simulink model "FOC_SMPMSM_SPWM"  (R2020b)
settings: Solver=FixedStepDiscrete  StartTime=0.0  StopTime=2  RelTol=1e-3
undefined symbols (not defined in the file): Kp_speed, Lq, PM_flux, pp, Rs
libraries: powerlib x23, simulink x5, pid_lib x3, powerlib_meascontrol x1
settings Model: SimulationMode=accelerator  Creator=ryusl  LastModifiedBy=90554
settings DataIOCC: SaveFormat=Array  ReturnWorkspaceOutputs=off
settings SFSimCC: CustomCodeUndefinedFunction=UseInterfaceOnly

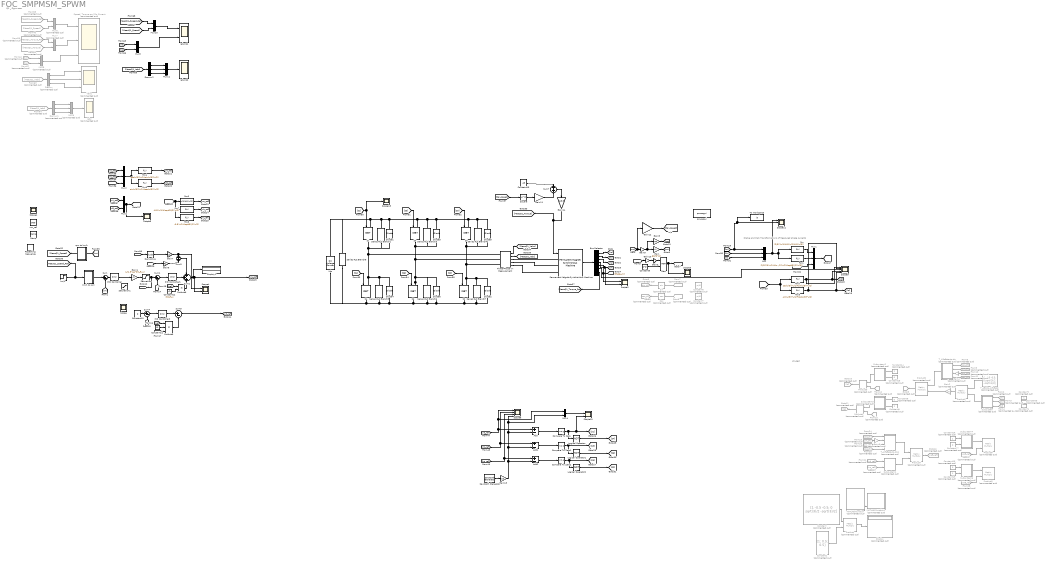
== system FOC_SMPMSM_SPWM ==
  note: Q1 _ Figures
  note: Unused
  note: Clarke and Park Transformations of Measured phase currents
  Add : Sum  Inputs=+-
  Add1 : Sum  Inputs=+-
  Add2 : Sum  Inputs=+-
  Bus Selector : BusSelector  OutputSignals=Stator current is_a (A),Stator current is_b (A),Stator current is_c (A),Rotor speed wm (rad/s),Rotor angle thetam (rad),Stator current is_d (A),Electromagnetic torque Te (N*m)
  Compare To Zero : simulink/Logic and Bit Operations/Compare To Zero  relop=>=  OutDataTypeStr=boolean
  Compare To Zero1 : simulink/Logic and Bit Operations/Compare To Zero  relop=>=  OutDataTypeStr=boolean
  Compare To Zero2 : simulink/Logic and Bit Operations/Compare To Zero  relop=>=  OutDataTypeStr=boolean
  Constant : Constant  Commented=on  Value=[1 -0.5 -0.5; 0 sqrt(3)/2 -sqrt(3)/2]  VectorParams1D=off
  Constant1 : Constant  Commented=on  Value=[1; 0.5; 0.5]  VectorParams1D=off
  Constant10 : Constant  Value=0
  Constant11 : Constant  Value=Lq
  Constant12 : Constant  Value=PM_flux
  Constant13 : Constant  Value=45
  Constant{2,9,14,16,19} (5 alike) : Constant  Commented=on
  Constant{8,15,17..18} (4 alike) : Constant  Commented=on  Value=0
  Constant3 : Constant  Commented=on  Value=-0.5
  Constant4 : Constant  Commented=on  Value=-0.5
  Constant5 : Constant  Value=2*pi
  Constant6 : Constant  Commented=on  Value=pi/6
  Constant7 : Constant  Commented=on  Value=pi/6
  Cos : Trigonometry  Commented=on  Operator=cos
  Demux : Demux  Commented=on  Outputs=3
  Demux1 : Demux  Commented=on  Outputs=3
  Demux2 : Demux  Outputs=3
  Derivative : Derivative
  Diode{1..6} (6 alike) : powerlib/Power Electronics/Diode  Ron=0.001  Lon=0  Vf=0.8  IC=0  UseSnubber=0  Rs=inf  Cs=0  Measurements=off
  Display : Display  Commented=on
  Display1 : Display
  Fcn : Fcn  Expr=(2/3)*(u(1)-0.5*u(2)-0.5*u(3))
  Fcn1 : Fcn  Expr=(2/3)*(0*u(1)+(sqrt(3)/2)*u(2)-(sqrt(3)/2)*u(3))
  Fcn2 : Fcn  Expr=cos(u(3))*u(1)+sin(u(3))*u(2)
  Fcn3 : Fcn  Expr=-sin(u(3))*u(1)+cos(u(3))*u(2)
  Fcn4 : Fcn  Expr=cos(u(3))*u(1)-sin(u(3))*u(2)
  Fcn5 : Fcn  Expr=sin(u(3))*u(1)+cos(u(3))*u(2)
  Fcn6 : Fcn  Expr=u(1)+0*u(2)
  Fcn7 : Fcn  Expr=-0.5*u(1)+(sqrt(3)/2)*u(2)
  Fcn8 : Fcn  Expr=-0.5*u(1)-(sqrt(3)/2)*u(2)
  From{9..10,23,26} (4 alike) : From  Commented=on  GotoTag=sin_th
  From{8,11,24..25} (4 alike) : From  Commented=on  GotoTag=cos_th
  From12 : From  Commented=on  GotoTag=idq
  From13 : From  Commented=on  GotoTag=idq
  From2 : From  Commented=on  GotoTag=ia
  From21 : From  Commented=on  GotoTag=vd_ref
  From22 : From  Commented=on  GotoTag=vq_ref
  From27 : From  Commented=on  GotoTag=vaB_ref
  From28 : From  Commented=on  GotoTag=vaB_ref
  From3 : From  Commented=on  GotoTag=ib
  From4 : From  Commented=on  GotoTag=ic
  From40 : From  Commented=on  GotoTag=MeasQ1_Speed
  From58 : From  Commented=on  GotoTag=MeasQ1_Speed_Ref
  From59 : From  Commented=on  GotoTag=MeasQ1_Torque_Ref
  From6 : From  Commented=on  GotoTag=theta_e
  From60 : From  Commented=on  GotoTag=MeasQ1_Torque
  From61 : From  Commented=on  GotoTag=id
  From62 : From  Commented=on  GotoTag=iq
  From63 : From  Commented=on  GotoTag=MeasQ1_Vabc
  From64 : From  Commented=on  GotoTag=MeasQ1_Iabc
  From7 : From  Commented=on  GotoTag=theta_e
  Gain : Gain  Gain=60/(2*pi)
  Gain1 : Gain  Gain=1/(1.5*pp*PM_flux)
  Gain10 : Gain
  Gain11 : Gain  Gain=0.105
  Gain12 : Gain  Gain=0.3/8.5
  Gain13 : Gain  Gain=210
  Gain14 : Gain  Gain=1/8.5
  Gain2 : Gain  Commented=on  Gain=2/3
  Gain3 : Gain  Gain=pp
  Gain4 : Gain  Commented=on  Gain=-1
  Gain5 : Gain  Gain=pp
  Gain6 : Gain  Gain=Rs
  Gain7 : Gain  Gain=Lq
  Gain8 : Gain  Commented=on  Gain=-1
  Gain9 : Gain
  Goto10 : Goto  Commented=on  GotoTag=id
  Goto11 : Goto  Commented=on  GotoTag=iq
  Goto16 : Goto  Commented=on  GotoTag=vaB_ref
  Goto6 : Goto  Commented=on  GotoTag=cos_th
  Goto8 : Goto  Commented=on  GotoTag=sin_th
  Goto9 : Goto  Commented=on  GotoTag=idq
  Iabc : Scope  Commented=on
  Iabc Q1 : Scope  NumInputPorts=2
  Iabc Q2 : Scope
  Logical Operator : Logic  Operator=NOT  AllPortsSameDT=off  OutDataTypeStr=boolean
  Logical Operator1 : Logic  Operator=NOT  AllPortsSameDT=off  OutDataTypeStr=boolean
  Logical Operator2 : Logic  Operator=NOT  AllPortsSameDT=off  OutDataTypeStr=boolean
  MATLAB Function : MATLAB Function  Commented=on  TreatAsAtomicUnit=on
  MATLAB Function1 : MATLAB Function  Commented=on  TreatAsAtomicUnit=on
  Mux{,1..2,11} (4 alike) : Mux  Inputs=3
  Mux{3..4,8,10} (4 alike) : Mux  Inputs=2
  Mux5 : Mux  Commented=on  Inputs=2
  Mux6 : Mux  Commented=on  Inputs=2
  Mux7 : Mux  Commented=on  Inputs=2
  Mux9 : Mux  Commented=on  Inputs=3
  PID Controller : pid_lib/PID Controller  Controller=PI  Form=Parallel  TimeDomain=Discrete-time  UseExternalTs=off  SampleTime=-1  IntegratorMethod=Forward Euler  FilterMethod=Forward Euler  ControllerParametersSource=internal  P=Kp_speed  I=2  D=0  UseFilter=on  N=100  TunerSelectOption=Transfer Function Based (PID Tuner App)  InitialConditionSource=internal  InitialConditionForIntegrator=0  InitialConditionForFilter=0  DifferentiatorICPrevScaledInput=0  ExternalReset=none  TrackingMode=off  Kt=1  LimitOutput=off  SatLimitsSource=internal  UpperSaturationLimit=inf  LowerSaturationLimit=-inf  LinearizeAsGain=on  AntiWindupMode=none  Kb=1  POutMin=[]  POutMax=[]  IOutMin=[]  IOutMax=[]  DOutMin=[]  DOutMax=[]  NOutMin=[]  NOutMax=[]  SumOutMin=[]  SumOutMax=[]  SaturationOutMin=[]  SaturationOutMax=[]  PParamMin=[]  PParamMax=[]  IParamMin=[]  IParamMax=[]  DParamMin=[]  DParamMax=[]  NParamMin=[]  NParamMax=[]  KbParamMin=[]  KbParamMax=[]  KtParamMin=[]  KtParamMax=[]  KbOutMin=[]  KbOutMax=[]  KtOutMin=[]  KtOutMax=[]  IntegratorOutMin=[]  IntegratorOutMax=[]  FilterOutMin=[]  FilterOutMax=[]  SumI1OutMin=[]  SumI1OutMax=[]  SumI2OutMin=[]  SumI2OutMax=[]  SumI3OutMin=[]  SumI3OutMax=[]  SumI4OutMin=[]  SumI4OutMax=[]  SumDOutMin=[]  SumDOutMax=[]  DifferentiatorOutMin=[]  DifferentiatorOutMax=[]  FilterDiffOutCoefMin=[]  FilterDiffOutCoefMax=[]  ReciprocalOutMin=[]  ReciprocalOutMax=[]  SumDenOutMin=[]  SumDenOutMax=[]  SumNumOutMin=[]  SumNumOutMax=[]  DivideOutMin=[]  DivideOutMax=[]  UdiffTsProdOutMin=[]  UdiffTsProdOutMax=[]  NTsProdOutMin=[]  NTsProdOutMax=[]  UintegralTsProdOutMin=[]  UintegralTsProdOutMax=[]  UngainTsProdOutMin=[]  UngainTsProdOutMax=[]  IntegratorContinuousStateAttributes=''  IntegratorStateMustResolveToSignalObject=off  IntegratorRTWStateStorageClass=Auto  FilterContinuousStateAttributes=''  FilterStateMustResolveToSignalObject=off  FilterRTWStateStorageClass=Auto  ParallelPVariant=InternalParameters  IdealPVariant=Disabled  IVariant=InternalParameters  DVariant=Disabled  IntegratorVariant=Discrete  SatVariant=Disabled  AWVariant=Passthrough  PCopyVariant=Disabled  TRVariant=Disabled  FdbkBlocksVariant=Forward  IdealPFdbkVariant=Disabled  SatFdbkVariant=Disabled  DerivativeFilterVariant=Disabled  NVariant=Disabled  NCopyVariant=Disabled_SignalSpec  FilterICVariant=Disabled  IntegratorICVariant=InternalICs  ExternalResetVariant=Disabled  TRSumVariant=Passthrough  SumFdbkVariant=Disabled  SumVariant=Sum_PI  TsampFilterVariant=InternalTs  TsampNgainVariant=Passthrough  TsampIntegralVariant=Passthrough  ExternalSaturationOutDataTypeStr=Inherit: Same as second input
  PID Controller1 : pid_lib/PID Controller  Controller=PI  Form=Parallel  TimeDomain=Discrete-time  UseExternalTs=off  SampleTime=-1  IntegratorMethod=Forward Euler  FilterMethod=Forward Euler  ControllerParametersSource=internal  P=10  I=1  D=0  UseFilter=on  N=100  TunerSelectOption=Transfer Function Based (PID Tuner App)  InitialConditionSource=internal  InitialConditionForIntegrator=0  InitialConditionForFilter=0  DifferentiatorICPrevScaledInput=0  ExternalReset=none  TrackingMode=off  Kt=1  LimitOutput=off  SatLimitsSource=internal  UpperSaturationLimit=inf  LowerSaturationLimit=-inf  LinearizeAsGain=on  AntiWindupMode=none  Kb=1  POutMin=[]  POutMax=[]  IOutMin=[]  IOutMax=[]  DOutMin=[]  DOutMax=[]  NOutMin=[]  NOutMax=[]  SumOutMin=[]  SumOutMax=[]  SaturationOutMin=[]  SaturationOutMax=[]  PParamMin=[]  PParamMax=[]  IParamMin=[]  IParamMax=[]  DParamMin=[]  DParamMax=[]  NParamMin=[]  NParamMax=[]  KbParamMin=[]  KbParamMax=[]  KtParamMin=[]  KtParamMax=[]  KbOutMin=[]  KbOutMax=[]  KtOutMin=[]  KtOutMax=[]  IntegratorOutMin=[]  IntegratorOutMax=[]  FilterOutMin=[]  FilterOutMax=[]  SumI1OutMin=[]  SumI1OutMax=[]  SumI2OutMin=[]  SumI2OutMax=[]  SumI3OutMin=[]  SumI3OutMax=[]  SumI4OutMin=[]  SumI4OutMax=[]  SumDOutMin=[]  SumDOutMax=[]  DifferentiatorOutMin=[]  DifferentiatorOutMax=[]  FilterDiffOutCoefMin=[]  FilterDiffOutCoefMax=[]  ReciprocalOutMin=[]  ReciprocalOutMax=[]  SumDenOutMin=[]  SumDenOutMax=[]  SumNumOutMin=[]  SumNumOutMax=[]  DivideOutMin=[]  DivideOutMax=[]  UdiffTsProdOutMin=[]  UdiffTsProdOutMax=[]  NTsProdOutMin=[]  NTsProdOutMax=[]  UintegralTsProdOutMin=[]  UintegralTsProdOutMax=[]  UngainTsProdOutMin=[]  UngainTsProdOutMax=[]  IntegratorContinuousStateAttributes=''  IntegratorStateMustResolveToSignalObject=off  IntegratorRTWStateStorageClass=Auto  FilterContinuousStateAttributes=''  FilterStateMustResolveToSignalObject=off  FilterRTWStateStorageClass=Auto  ParallelPVariant=InternalParameters  IdealPVariant=Disabled  IVariant=InternalParameters  DVariant=Disabled  IntegratorVariant=Discrete  SatVariant=Disabled  AWVariant=Passthrough  PCopyVariant=Disabled  TRVariant=Disabled  FdbkBlocksVariant=Forward  IdealPFdbkVariant=Disabled  SatFdbkVariant=Disabled  DerivativeFilterVariant=Disabled  NVariant=Disabled  NCopyVariant=Disabled_SignalSpec  FilterICVariant=Disabled  IntegratorICVariant=InternalICs  ExternalResetVariant=Disabled  TRSumVariant=Passthrough  SumFdbkVariant=Disabled  SumVariant=Sum_PI  TsampFilterVariant=InternalTs  TsampNgainVariant=Passthrough  TsampIntegralVariant=Passthrough  ExternalSaturationOutDataTypeStr=Inherit: Same as second input
  PID Controller2 : pid_lib/PID Controller  Controller=PI  Form=Parallel  TimeDomain=Discrete-time  UseExternalTs=off  SampleTime=-1  IntegratorMethod=Forward Euler  FilterMethod=Forward Euler  ControllerParametersSource=internal  P=10  I=1  D=0  UseFilter=on  N=100  TunerSelectOption=Transfer Function Based (PID Tuner App)  InitialConditionSource=internal  InitialConditionForIntegrator=0  InitialConditionForFilter=0  DifferentiatorICPrevScaledInput=0  ExternalReset=none  TrackingMode=off  Kt=1  LimitOutput=off  SatLimitsSource=internal  UpperSaturationLimit=inf  LowerSaturationLimit=-inf  LinearizeAsGain=on  AntiWindupMode=none  Kb=1  POutMin=[]  POutMax=[]  IOutMin=[]  IOutMax=[]  DOutMin=[]  DOutMax=[]  NOutMin=[]  NOutMax=[]  SumOutMin=[]  SumOutMax=[]  SaturationOutMin=[]  SaturationOutMax=[]  PParamMin=[]  PParamMax=[]  IParamMin=[]  IParamMax=[]  DParamMin=[]  DParamMax=[]  NParamMin=[]  NParamMax=[]  KbParamMin=[]  KbParamMax=[]  KtParamMin=[]  KtParamMax=[]  KbOutMin=[]  KbOutMax=[]  KtOutMin=[]  KtOutMax=[]  IntegratorOutMin=[]  IntegratorOutMax=[]  FilterOutMin=[]  FilterOutMax=[]  SumI1OutMin=[]  SumI1OutMax=[]  SumI2OutMin=[]  SumI2OutMax=[]  SumI3OutMin=[]  SumI3OutMax=[]  SumI4OutMin=[]  SumI4OutMax=[]  SumDOutMin=[]  SumDOutMax=[]  DifferentiatorOutMin=[]  DifferentiatorOutMax=[]  FilterDiffOutCoefMin=[]  FilterDiffOutCoefMax=[]  ReciprocalOutMin=[]  ReciprocalOutMax=[]  SumDenOutMin=[]  SumDenOutMax=[]  SumNumOutMin=[]  SumNumOutMax=[]  DivideOutMin=[]  DivideOutMax=[]  UdiffTsProdOutMin=[]  UdiffTsProdOutMax=[]  NTsProdOutMin=[]  NTsProdOutMax=[]  UintegralTsProdOutMin=[]  UintegralTsProdOutMax=[]  UngainTsProdOutMin=[]  UngainTsProdOutMax=[]  IntegratorContinuousStateAttributes=''  IntegratorStateMustResolveToSignalObject=off  IntegratorRTWStateStorageClass=Auto  FilterContinuousStateAttributes=''  FilterStateMustResolveToSignalObject=off  FilterRTWStateStorageClass=Auto  ParallelPVariant=InternalParameters  IdealPVariant=Disabled  IVariant=InternalParameters  DVariant=Disabled  IntegratorVariant=Discrete  SatVariant=Disabled  AWVariant=Passthrough  PCopyVariant=Disabled  TRVariant=Disabled  FdbkBlocksVariant=Forward  IdealPFdbkVariant=Disabled  SatFdbkVariant=Disabled  DerivativeFilterVariant=Disabled  NVariant=Disabled  NCopyVariant=Disabled_SignalSpec  FilterICVariant=Disabled  IntegratorICVariant=InternalICs  ExternalResetVariant=Disabled  TRSumVariant=Passthrough  SumFdbkVariant=Disabled  SumVariant=Sum_PI  TsampFilterVariant=InternalTs  TsampNgainVariant=Passthrough  TsampIntegralVariant=Passthrough  ExternalSaturationOutDataTypeStr=Inherit: Same as second input
  Permanent Magnet Synchronous Machine : powerlib/Machines/Permanent Magnet Synchronous Machine  NbPhases=3  FluxDistribution=Sinusoidal  RotorType=Round  MechanicalLoad=Torque Tm  PresetModel=No  ShowDetailedParameters=on  MeasurementBus=off  Resistance=Rs  Inductance=8.5e-3  dqInductances=[8.5e-3,8.5e-3]  La=Ld  MachineConstant=Flux linkage established by magnets (V.s)  Flux=PM_flux  VoltageCst=79.8072  TorqueCst=0.66  Flat=120  Mechanical=[2.4232 0 4 0]  PolePairs=4  InitialConditions=[(40*8.5)/(3.6*0.3),0, 0,0]  InitialConditions5ph=[0 0 0 0 0 0]  RefAngle=Aligned with phase A axis (original Park)  IterativeDiscreteModel=Trapezoidal non iterative  TsBlock=1e-6  TsPowergui=0
  Product{,1..4,7..9} (8 alike) : Product  Commented=on  Multiplication=Matrix(*)
  Product5 : Product  Inputs=3
  Product6 : Product
  Ramp : simulink/Sources/Ramp  slope=1000  start=0  InitialOutput=0
  Rem : Math  Operator=rem  SignedPower=on  SaturateOnIntegerOverflow=on
  Repeating Sequence : simulink/Sources/Repeating Sequence  rep_seq_t=[0 0.5 0.7 0.7001 1.2]  rep_seq_y=[0 35 35 40 40]
  S{1..6} (6 alike) : powerlib/Power Electronics/IGBT  Ron=0.001  Lon=0  Vf=1  Tf=1e-6  Tt=2e-6  IC=0  Rs=1e5  Cs=inf  Measurements=off
  Saturation : Saturate  UpperLimit=530  LowerLimit=-530
  Saturation1 : Saturate  UpperLimit=350  LowerLimit=-350
  Sawtooth Generator : powerlib_meascontrol/Pulse & Signal Generators/Sawtooth Generator  Freq=20e3  Phase=180  Ts=0
  Scope{,2,4,10} (4 alike) : Scope  NumInputPorts=2
  Scope{1,3,8,13} (4 alike) : Scope
  Scope11 : Scope  NumInputPorts=3
  Scope6 : Scope  NumInputPorts=4
  Scope9 : Scope  NumInputPorts=5
  Series RLC Branch{1,3..7} (6 alike) : powerlib/Elements/Series RLC Branch  LConnTagsString=__new0  RConnTagsString=__new0  BranchType=RC  Resistance=100  Inductance=1e-3  SetiL0=off  InitialCurrent=0  Capacitance=1e-12  Setx0=off  InitialVoltage=0  Measurements=None
  Series RLC Branch8 : powerlib/Elements/Series RLC Branch  LConnTagsString=__new0  RConnTagsString=__new0  BranchType=RC  Resistance=1e-3  Inductance=1e-3  SetiL0=off  InitialCurrent=0  Capacitance=220e-6  Setx0=off  InitialVoltage=0  Measurements=None
  Sin : Trigonometry  Commented=on
  "Speed, Torque and Dq Current" : Scope  Commented=on  NumInputPorts=3
  Square : Math  Operator=square  SignedPower=on  SaturateOnIntegerOverflow=on
  Subsystem : Subsystem  Commented=on
  Subsystem1 : Subsystem  Commented=on
  Subsystem2 : Subsystem  Commented=on
  Subsystem3 : Subsystem  Commented=on
  Subsystem4 : Subsystem  Commented=on
  Subsystem6 : Subsystem  Commented=on
  Sum{,1,4..5} (4 alike) : Sum  Inputs=|+-
  Sum2 : Sum  Inputs=+|+|+
  Sum3 : Sum  Inputs=+|+
  Sum7 : Sum  Inputs=+|+
  T_ABC-to-AlfaBeta : Constant  Commented=on  Value=[1 -0.5 -0.5; 0 sqrt(3)/2 -sqrt(3)/2]  VectorParams1D=off
  T_AlfaBeta-to-dq : Subsystem  Commented=on
  T_AlfaBeta-to-dq1 : Subsystem  Commented=on
  Three-Phase V-I Measurement : powerlib/Measurements/Three-Phase V-I Measurement  VoltageMeasurement=phase-to-phase  SetLabelV=off  LabelV=Vabc  Vpu=off  VpuLL=off  CurrentMeasurement=yes  SetLabelI=off  LabelI=Iabc  Ipu=off  Pbase=100e6  Vbase=500e3  OutputType=Complex  PhasorSimulation=off  PSBequivalent=0
  To Workspace : ToWorkspace  VariableName=ia  SaveFormat=Structure With Time  SampleTime=1e-5
  Vabc : Scope  Commented=on  NumInputPorts=3
  Vdc : powerlib/Electrical Sources/DC Voltage Source  Amplitude=420  Measurements=Voltage
  km/h : Step  Before=40  After=-8  SampleTime=0
  km/h to rpm : Subsystem
  nm_ref : Constant  Value=500
  powergui : powerlib/powergui  Priority=1  SimulationMode=Discrete  SampleTime=1e-6  frequency=60  Iterations=50  frequencyindice=0  Pbase=100e6  ErrMax=1e-4  UnitsV=kV  UnitsW=MW  buscounter=0  FunctionMessages=off  echomessages=off  EnableUseOfTLC=off  CurrentSourceSwitches=off  DisableSnubberDevices=off  DisableRonSwitches=off  DisableVfSwitches=off  DisplayEquations=off  AutomaticDiscreteSolvers=off  SolverType=Tustin/Backward Euler (TBE)  Interpol=off  ExternalGateDelay=off  methode=off  Ts=100  x0status=blocks  SPID=on  SwTol=0  HookPort=off  NonlinearTolerance=0  nMaxIteration=15  ContinueOnMaxIteration=off  RestoreLinks=warning  ResistiveCurrentMeasurement=off  Frange=[0:2:500]  Ylog=off  Xlog=on  ShowGrid=off  save=off  variable=ZData  structure=ia  ZoomFFT=off  StartTime=0.472  cycles=1  DisplayStyle=1  fundamental=64  FreqAxis=off  MaxFrequency=1000  frequencyindicesteady=1  RmsSteady=1  display=off
  rpm to km/h : Subsystem
  wires:
  Constant/1 -> Product/1
  Constant1/1 -> Product/2
  Product/1 -> Display/1
  Permanent Magnet Synchronous Machine/1 -> Bus Selector/1
  Bus Selector/1 -> [ia]  "<Stator current is_a (A)>"
  Bus Selector/2 -> [ib]  "<Stator current is_b (A)>"
  Bus Selector/3 -> [ic]  "<Stator current is_c (A)>"
  Bus Selector/4 -> Scope2/2, [wm]  "<Rotor speed wm (rad/s)>"
  Bus Selector/5 -> Scope2/1, [theta_m]  "<Rotor angle thetam (rad)>"
  Gain/1 -> [nm]
  Sum/1 -> PID Controller/1
  [nm] -> Sum/2
  T_ABC-to-AlfaBeta/1 -> Product1/1
  Subsystem/1(Matrix) -> Product1/2
  Product1/1 -> Gain2/1
  Constant5/1 -> Rem/2
  Gain3/1 -> Rem/1
  Rem/1 -> Scope3/1, [theta_e]
  Cos/1 -> Goto6/1
  Sin/1 -> Goto8/1
  Gain4/1 -> T_AlfaBeta-to-dq/3(M21)
  From8/1 -> T_AlfaBeta-to-dq/1(M11)
  From9/1 -> T_AlfaBeta-to-dq/2(M12)
  From10/1 -> Gain4/1
  From11/1 -> T_AlfaBeta-to-dq/4("M22 ")
  Gain2/1 -> Product2/2
  T_AlfaBeta-to-dq/1(Matrix) -> Product2/1
  Product2/1 -> Goto9/1
  From12/1 -> Product3/2
  Product3/1 -> Goto10/1
  Product4/1 -> Goto11/1
  [iq] -> Sum1/2
  Sum1/1 -> PID Controller1/1
  PID Controller1/1 -> Sum2/2
  Gain5/1 -> [we]
  Sum4/1 -> PID Controller2/1
  [id] -> Sum4/2
  Constant10/1 -> Sum4/1
  [iq_ref] -> Product5/3
  Constant11/1 -> Product5/2
  [we] -> Product5/1
  PID Controller2/1 -> Sum5/1
  [we] -> Product6/1
  Constant12/1 -> Product6/2
  [iq_ref] -> Gain6/1
  Gain6/1 -> Sum3/2
  Gain7/1 -> Scope4/1, Sum3/1
  From22/1 -> Subsystem1/2(M21)
  From21/1 -> Subsystem1/1(M11)
  Constant14/1 -> Subsystem2/1(M11)
  Constant15/1 -> Subsystem2/2(M21)
  Subsystem2/1(Matrix) -> Product3/1
  Constant8/1 -> Subsystem3/1(M11)
  Constant9/1 -> Subsystem3/2(M21)
  Subsystem3/1(Matrix) -> Product4/1
  From13/1 -> Product4/2
  From23/1 -> Gain8/1
  Gain8/1 -> T_AlfaBeta-to-dq1/2(M12)
  From24/1 -> T_AlfaBeta-to-dq1/1(M11)
  From26/1 -> T_AlfaBeta-to-dq1/3(M21)
  From25/1 -> T_AlfaBeta-to-dq1/4("M22 ")
  T_AlfaBeta-to-dq1/1(Matrix) -> Product7/1
  Subsystem1/1(Matrix) -> Product7/2
  Constant17/1 -> Subsystem4/2(M21)
  Constant16/1 -> Subsystem4/1(M11)
  Subsystem4/1(Matrix) -> Product8/1
  From27/1 -> Product8/2
  From28/1 -> Product9/2
  Subsystem6/1(Matrix) -> Product9/1
  Constant18/1 -> Subsystem6/1(M11)
  Constant19/1 -> Subsystem6/2(M21)
  Product7/1 -> Goto16/1
  From7/1 -> Sin/1
  From6/1 -> Cos/1
  From2/1 -> Subsystem/1(M11)
  From3/1 -> Subsystem/2(M21)
  From4/1 -> Subsystem/3(M31)
  Gain1/1 -> Saturation/1
  Saturation/1 -> [iq_ref], Sum1/1
  [wm] -> Gain12/1, Gain9/1
  Gain9/1 -> Gain5/1, Gain/1
  [theta_m] -> Gain10/1
  Gain10/1 -> Gain3/1
  Fcn/1 -> Mux1/1  "iAlfa"
  Fcn1/1 -> Mux1/2  "iBeta"
  [theta_e] -> Mux1/3
  Mux1/1 -> [iaB_th]
  [iaB_th] -> Fcn3/1, Fcn2/1
  Fcn2/1 -> Scope9/4, [id], Scope9/1  "id"
  Fcn3/1 -> [iq], Scope9/5, Scope9/2  "iq"
  [vd_ref] -> Mux2/1
  [vq_ref] -> Mux2/2
  [theta_e] -> Mux2/3
  Mux2/1 -> Fcn5/1, Fcn4/1
  Fcn5/1 -> [vB_ref]  "vBeta_ref"
  Fcn4/1 -> [vA_ref]  "vAlfa_ref"
  [vA_ref] -> Mux3/1
  [vB_ref] -> Mux3/2
  Mux3/1 -> Scope8/1, [vaB_ref]
  Bus Selector/6 -> Scope9/3  "<Stator current is_d (A)>"
  [vaB_ref] -> Fcn8/1, Fcn7/1, Fcn6/1
  Fcn6/1 -> [va_ref]  "va_ref"
  Fcn7/1 -> [vb_ref]  "vb_ref"
  Fcn8/1 -> [vc_ref]  "vc_ref"
  MATLAB Function/3(iz_aB) -> MATLAB Function1/3(theta)
  Mux4/1 -> Scope10/1
  Compare To Zero2/1 -> Logical Operator2/1, [S5]
  Compare To Zero/1 -> Logical Operator/1, [S1], Scope10/2
  Logical Operator/1 -> [S4]
  Compare To Zero1/1 -> Logical Operator1/1, [S3]
  Add1/1 -> Compare To Zero1/1
  Logical Operator2/1 -> [S2]
  Logical Operator1/1 -> [S6]
  [va_ref] -> Add/1, Scope6/1, Mux4/1
  [vb_ref] -> Scope6/2, Add1/1
  [vc_ref] -> Add2/1, Scope6/3
  Sawtooth Generator/1 -> Gain13/1
  Add/1 -> Compare To Zero/1
  Add2/1 -> Compare To Zero2/1
  Gain13/1 -> Add2/2, Add1/2, Add/2, Mux4/2, Scope6/4
  Sum3/1 -> Sum2/1
  Product6/1 -> Sum2/3
  Product5/1 -> Sum5/2
  Mux/1 -> Scope11/1, Fcn1/1, Fcn/1
  Sum2/1 -> [vq_ref], Scope4/2, Display1/1
  [S4] -> S4/1
  [S6] -> S6/1
  [S3] -> S3/1
  [S5] -> S5/1
  [S2] -> S2/1
  [S1] -> S1/1, Scope13/1
  [ia] -> Mux/1, Scope11/2, To Workspace/1
  [ib] -> Mux/2
  [ic] -> Mux/3
  Sum5/1 -> [vd_ref]
  Derivative/1 -> Gain7/1
  [iq_ref] -> Derivative/1
  km/h to rpm/1(Out1) -> Sum/1
  Sum7/1 -> Gain14/1
  [Car_speed] -> Square/1
  Square/1 -> Gain11/1
  Constant13/1 -> Sum7/1
  Gain11/1 -> Sum7/2
  Gain12/1 -> [Car_speed]
  rpm to km/h/1(Out1) -> [MeasQ1_Speed]
  [nm] -> rpm to km/h/1(In1)
  From58/1 -> Mux6/1  "Speed*"
  From40/1 -> Mux6/2  "Speed"
  From59/1 -> Mux7/1  "Motor Torque"
  From60/1 -> Mux7/2  "Load Torque"
  From61/1 -> Mux5/1  "id"
  From62/1 -> Mux5/2  "iq"
  Mux6/1 -> "Speed, Torque and Dq Current"/1
  Mux7/1 -> "Speed, Torque and Dq Current"/2
  Mux5/1 -> "Speed, Torque and Dq Current"/3
  Three-Phase V-I Measurement/1 -> [MeasQ1_Vabc]
  Three-Phase V-I Measurement/2 -> [MeasQ1_Iabc]
  From63/1 -> Demux/1
  Demux/1 -> Vabc/1  "Va"
  Demux/2 -> Vabc/2  "Vb"
  Demux/3 -> Vabc/3  "Vc"
  Demux1/3 -> Mux9/3  "Ic"
  Demux1/1 -> Mux9/1  "Ia"
  Demux1/2 -> Mux9/2  "Ib"
  From64/1 -> Demux1/1
  Mux9/1 -> Iabc/1
  km/h/1 -> [MeasQ1_Speed_Ref], km/h to rpm/1(In1)
  Mux8/1 -> Iabc Q1/2
  [id] -> Mux8/1  "id"
  [iq] -> Mux8/2  "iq"
  Mux10/1 -> Iabc Q1/1
  [MeasQ1_Speed_Ref] -> Mux10/1  "Speed*"
  [MeasQ1_Speed] -> Mux10/2  "Speed"
  Demux2/1 -> Mux11/1  "Ia"
  Demux2/3 -> Mux11/3  "Ic"
  [MeasQ1_Iabc] -> Demux2/1
  Demux2/2 -> Mux11/2  "Ib"
  Mux11/1 -> Iabc Q2/1
  Gain14/1 -> [MeasQ1_Torque], Permanent Magnet Synchronous Machine/1
  PID Controller/1 -> Gain1/1
  Bus Selector/7 -> [MeasQ1_Torque_Ref]  "<Electromagnetic torque Te (N*m)>"
  connections:
  S6/LConn1 -- Three-Phase V-I Measurement/LConn2 -- Series RLC Branch3/RConn1 -- Diode3/LConn1 -- S3/RConn1 -- Diode6/RConn1 -- Series RLC Branch6/LConn1
  S5/LConn1 -- Series RLC Branch3/LConn1 -- Series RLC Branch1/LConn1 -- Series RLC Branch8/LConn1 -- Vdc/RConn1 -- S1/LConn1 -- Diode1/RConn1 -- S3/LConn1 -- Diode3/RConn1 -- Series RLC Branch4/LConn1 -- Diode5/RConn1
  Series RLC Branch6/RConn1 -- Series RLC Branch5/RConn1 -- Series RLC Branch8/RConn1 -- Vdc/LConn1 -- S4/RConn1 -- Diode4/LConn1 -- S6/RConn1 -- Diode6/LConn1 -- S2/RConn1 -- Diode2/LConn1 -- Series RLC Branch7/RConn1
  Diode2/RConn1 -- Series RLC Branch7/LConn1 -- Three-Phase V-I Measurement/LConn3 -- Diode5/LConn1 -- Series RLC Branch4/RConn1 -- S5/RConn1 -- S2/LConn1
  Diode4/RConn1 -- Series RLC Branch5/LConn1 -- S4/LConn1 -- Three-Phase V-I Measurement/LConn1 -- Series RLC Branch1/RConn1 -- Diode1/LConn1 -- S1/RConn1
  Three-Phase V-I Measurement/RConn1 -- Permanent Magnet Synchronous Machine/LConn1
  Three-Phase V-I Measurement/RConn2 -- Permanent Magnet Synchronous Machine/LConn2
  Three-Phase V-I Measurement/RConn3 -- Permanent Magnet Synchronous Machine/LConn3

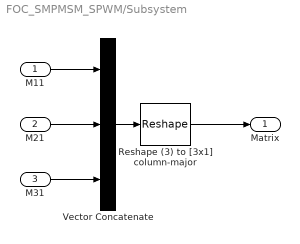
== system FOC_SMPMSM_SPWM/Subsystem ==
  M11 : Inport  PortDimensions=1
  M21 : Inport  Port=2  PortDimensions=1
  M31 : Inport  Port=3  PortDimensions=1
  Reshape (3) to [3x1] column-major : Reshape  OutputDimensionality=Customize  OutputDimensions=[3,1]
  Vector Concatenate : Concatenate  NumInputs=3
  Matrix : Outport  PortDimensions=[3 1]  VectorParamsAs1DForOutWhenUnconnected=off
  wires:
  M11/1 -> Vector Concatenate/1
  Vector Concatenate/1 -> Reshape (3) to [3x1] column-major/1
  M21/1 -> Vector Concatenate/2
  Reshape (3) to [3x1] column-major/1 -> Matrix/1
  M31/1 -> Vector Concatenate/3

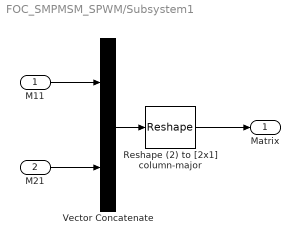
== system FOC_SMPMSM_SPWM/Subsystem1 ==
  M11 : Inport  PortDimensions=1
  M21 : Inport  Port=2  PortDimensions=1
  Reshape (2) to [2x1] column-major : Reshape  OutputDimensionality=Customize  OutputDimensions=[2,1]
  Vector Concatenate : Concatenate
  Matrix : Outport  PortDimensions=[2 1]  VectorParamsAs1DForOutWhenUnconnected=off
  wires:
  Reshape (2) to [2x1] column-major/1 -> Matrix/1
  M21/1 -> Vector Concatenate/2
  Vector Concatenate/1 -> Reshape (2) to [2x1] column-major/1
  M11/1 -> Vector Concatenate/1

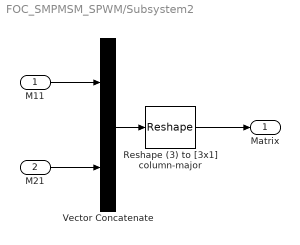
== system FOC_SMPMSM_SPWM/Subsystem2 ==
  M11 : Inport  PortDimensions=1
  M21 : Inport  Port=2  PortDimensions=1
  Reshape (3) to [3x1] column-major : Reshape  OutputDimensionality=Customize  OutputDimensions=[1,2]
  Vector Concatenate : Concatenate
  Matrix : Outport  PortDimensions=[1 2]  VectorParamsAs1DForOutWhenUnconnected=off
  wires:
  M11/1 -> Vector Concatenate/1
  Vector Concatenate/1 -> Reshape (3) to [3x1] column-major/1
  M21/1 -> Vector Concatenate/2
  Reshape (3) to [3x1] column-major/1 -> Matrix/1

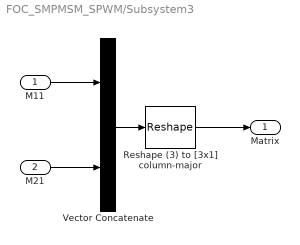
== system FOC_SMPMSM_SPWM/Subsystem3 ==
  M11 : Inport  PortDimensions=1
  M21 : Inport  Port=2  PortDimensions=1
  Reshape (3) to [3x1] column-major : Reshape  OutputDimensionality=Customize  OutputDimensions=[1,2]
  Vector Concatenate : Concatenate
  Matrix : Outport  PortDimensions=[1 2]  VectorParamsAs1DForOutWhenUnconnected=off
  wires:
  M11/1 -> Vector Concatenate/1
  Vector Concatenate/1 -> Reshape (3) to [3x1] column-major/1
  M21/1 -> Vector Concatenate/2
  Reshape (3) to [3x1] column-major/1 -> Matrix/1

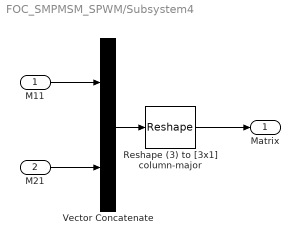
== system FOC_SMPMSM_SPWM/Subsystem4 ==
  M11 : Inport  PortDimensions=1
  M21 : Inport  Port=2  PortDimensions=1
  Reshape (3) to [3x1] column-major : Reshape  OutputDimensionality=Customize  OutputDimensions=[1,2]
  Vector Concatenate : Concatenate
  Matrix : Outport  PortDimensions=[1 2]  VectorParamsAs1DForOutWhenUnconnected=off
  wires:
  Reshape (3) to [3x1] column-major/1 -> Matrix/1
  M21/1 -> Vector Concatenate/2
  Vector Concatenate/1 -> Reshape (3) to [3x1] column-major/1
  M11/1 -> Vector Concatenate/1

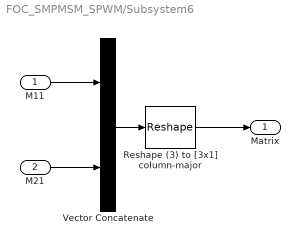
== system FOC_SMPMSM_SPWM/Subsystem6 ==
  M11 : Inport  PortDimensions=1
  M21 : Inport  Port=2  PortDimensions=1
  Reshape (3) to [3x1] column-major : Reshape  OutputDimensionality=Customize  OutputDimensions=[1,2]
  Vector Concatenate : Concatenate
  Matrix : Outport  PortDimensions=[1 2]  VectorParamsAs1DForOutWhenUnconnected=off
  wires:
  M11/1 -> Vector Concatenate/1
  Vector Concatenate/1 -> Reshape (3) to [3x1] column-major/1
  M21/1 -> Vector Concatenate/2
  Reshape (3) to [3x1] column-major/1 -> Matrix/1

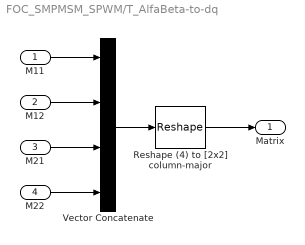
== system FOC_SMPMSM_SPWM/T_AlfaBeta-to-dq ==
  M11 : Inport  PortDimensions=1
  M12 : Inport  Port=2  PortDimensions=1
  M21 : Inport  Port=3  PortDimensions=1
  "M22 " : Inport  Port=4  PortDimensions=1
  Reshape (4) to [2x2] column-major : Reshape  OutputDimensionality=Customize  OutputDimensions=[2,2]
  Vector Concatenate : Concatenate  NumInputs=4
  Matrix : Outport  PortDimensions=[2 2]  VectorParamsAs1DForOutWhenUnconnected=off
  wires:
  M21/1 -> Vector Concatenate/3
  Reshape (4) to [2x2] column-major/1 -> Matrix/1
  M12/1 -> Vector Concatenate/2
  Vector Concatenate/1 -> Reshape (4) to [2x2] column-major/1
  M11/1 -> Vector Concatenate/1
  "M22 "/1 -> Vector Concatenate/4

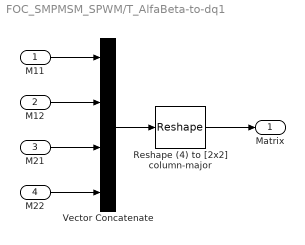
== system FOC_SMPMSM_SPWM/T_AlfaBeta-to-dq1 ==
  M11 : Inport  PortDimensions=1
  M12 : Inport  Port=2  PortDimensions=1
  M21 : Inport  Port=3  PortDimensions=1
  "M22 " : Inport  Port=4  PortDimensions=1
  Reshape (4) to [2x2] column-major : Reshape  OutputDimensionality=Customize  OutputDimensions=[2,2]
  Vector Concatenate : Concatenate  NumInputs=4
  Matrix : Outport  PortDimensions=[2 2]  VectorParamsAs1DForOutWhenUnconnected=off
  wires:
  M21/1 -> Vector Concatenate/3
  Reshape (4) to [2x2] column-major/1 -> Matrix/1
  M12/1 -> Vector Concatenate/2
  Vector Concatenate/1 -> Reshape (4) to [2x2] column-major/1
  M11/1 -> Vector Concatenate/1
  "M22 "/1 -> Vector Concatenate/4

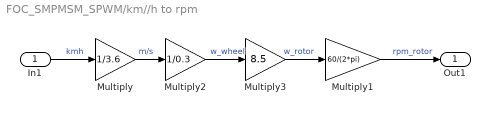
== system FOC_SMPMSM_SPWM/km//h to rpm ==
  In1 : Inport
  Multiply : Gain  Gain=1/3.6
  Multiply1 : Gain  Gain=60/(2*pi)
  Multiply2 : Gain  Gain=1/0.3
  Multiply3 : Gain  Gain=8.5
  Out1 : Outport
  wires:
  In1/1 -> Multiply/1  "kmh"
  Multiply1/1 -> Out1/1  "rpm_rotor"
  Multiply/1 -> Multiply2/1  "m/s"
  Multiply3/1 -> Multiply1/1  "w_rotor"
  Multiply2/1 -> Multiply3/1  "w_wheel"

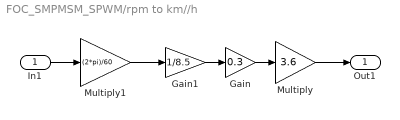
== system FOC_SMPMSM_SPWM/rpm to km//h ==
  In1 : Inport
  Gain : Gain  Gain=0.3
  Gain1 : Gain  Gain=1/8.5
  Multiply : Gain  Gain=3.6
  Multiply1 : Gain  Gain=(2*pi)/60
  Out1 : Outport
  wires:
  In1/1 -> Multiply1/1
  Multiply/1 -> Out1/1
  Gain/1 -> Multiply/1
  Multiply1/1 -> Gain1/1
  Gain1/1 -> Gain/1

== matlab function FOC_SMPMSM_SPWM/MATLAB Function1 ==
  data: ialfa input; id output; iB input; theta input; iq output
function [id,iq] = aB_dq(ialfa,iB,theta)
T_aB-dq = [cos(theta) sin(theta); -sin(theta) cos(theta)];
[id,iq] = T_ab-dq*[ialfa; iB];

== matlab function FOC_SMPMSM_SPWM/MATLAB Function ==
  data: ialfa output; ia input; ib input; ic input; iB output; iz_aB output
function [ialfa,iB,iz_aB] = abc_aB(ia,ib,ic)
T_abc_aB = (2/3).*[1 -0.5 -0.5; 0 sqrt(3)/2 -sqrt(3)/2; 0.5 0.5 0.5];
[ialfa,iB,iz_aB] = T_abc_aB*[ia; ib; ic];
